simulink model "dual_single_phase_parallel_inverter_r2024a"  (R2024a)
settings: Solver=ode23t  StartTime=0.0  StopTime=0.25  MaxStep=5e-6  RelTol=1e-4
model workspace (MAT data in the model file):
  Paux1_W = 1
  Paux2_W = 1
libraries: nesl_utility x41, fl_lib x39, ee_lib x31, simulink x6
(part 4 of 4)

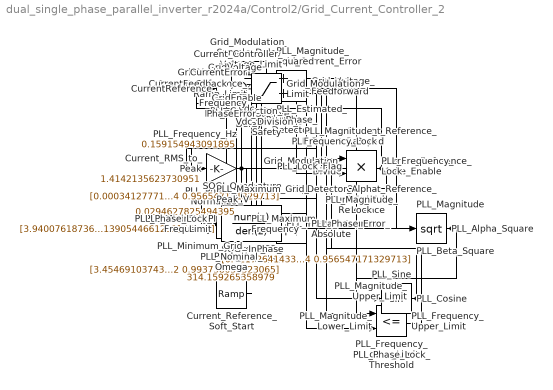
== system dual_single_phase_parallel_inverter_r2024a/Control2/Grid_Current_Controller_2 ==
  GridVoltage : Inport
  IrefRms : Inport  Port=2
  CurrentFeedback : Inport  Port=3
  Vdc : Inport  Port=4
  GridEnable : Inport  Port=5
  Current_Controller_Voltage_Limit : Saturate  UpperLimit=16  LowerLimit=-16
  Current_PR_Controller : DiscreteTransferFcn  Numerator=[3.45469103743655 -6.26042259834152 2.80882171809216]  Denominator=[1 -1.99275440474052 0.993738032323065]  SampleTime=1e-4
  Current_RMS_to_Peak : Gain  Gain=1.4142135623730951
  Current_Reference_Mode_Enable : Product
  Current_Reference_PLL_Lock : Product
  Current_Reference_Ramp_Limit : Saturate  UpperLimit=1  LowerLimit=0
  Current_Reference_Ramped : Product
  Current_Reference_Soft_Start : simulink/Sources/Ramp  slope=5  start=0  InitialOutput=0
  Current_Sine_Reference : Product
  Grid_Current_Error : Sum  Inputs=+-
  Grid_Modulation_Divide : Product  Inputs=*/
  Grid_Modulation_Limit : Saturate  UpperLimit=0.95  LowerLimit=-0.95
  Grid_Modulation_Sample_Delay : UnitDelay  SampleTime=1e-4  HasFrameUpgradeWarning=on
  Grid_Voltage_Feedforward : Sum
  PLL_Alpha_Square : Math  Operator=square
  PLL_Beta_Square : Math  Operator=square
  PLL_Correction_Limit : Saturate  UpperLimit=31.4159265359  LowerLimit=-31.4159265359
  PLL_Cosine : Trigonometry  Operator=cos
  PLL_Detector_Alpha : Product
  PLL_Detector_Beta : Product
  PLL_Estimated_Omega : Sum
  PLL_Frequency_Hz : Gain  Gain=0.159154943091895
  PLL_Frequency_Lock : Product
  PLL_Frequency_Lower_Limit : RelationalOperator  OutDataTypeStr=boolean  RndMeth=Simplest  InputSameDT=off
  PLL_Frequency_Upper_Limit : RelationalOperator  Operator=<=  OutDataTypeStr=boolean  RndMeth=Simplest  InputSameDT=off
  PLL_Lock_Flag : Product
  PLL_Magnitude : Math  Operator=sqrt
  PLL_Magnitude_Frequency_Lock : Product
  PLL_Magnitude_Lock : Product
  PLL_Magnitude_Lower_Limit : RelationalOperator  OutDataTypeStr=boolean  RndMeth=Simplest  InputSameDT=off
  PLL_Magnitude_Squared : Sum
  PLL_Magnitude_Upper_Limit : RelationalOperator  Operator=<=  OutDataTypeStr=boolean  RndMeth=Simplest  InputSameDT=off
  PLL_Maximum_Frequency : Constant  Value=50.5
  PLL_Maximum_Grid_Peak_V : Constant  Value=48
  PLL_Minimum_Frequency : Constant  Value=49.5
  PLL_Minimum_Grid_Peak_V : Constant  Value=20
  PLL_Nominal_Omega : Constant  Value=314.159265358979
  PLL_PI : DiscreteTransferFcn  Numerator=[3.94007618736156 -3.91390544661292]  Denominator=[1 -1]  SampleTime=1e-4
  PLL_Phase_Detector : Sum
  PLL_Phase_Error_Absolute : Abs  SaturateOnIntegerOverflow=off
  PLL_Phase_Lock_Limit : Constant  Value=0.05
  PLL_Phase_Lock_Threshold : RelationalOperator  Operator=<=  OutDataTypeStr=boolean  RndMeth=Simplest  InputSameDT=off
  PLL_Phase_Normalize : Gain  Gain=0.0294627825494395
  PLL_Sine : Trigonometry
  PLL_Theta_Integrator : DiscreteTransferFcn  Numerator=[1e-4 0]  Denominator=[1 -1]  SampleTime=1e-4
  PLL_Theta_Sample_Delay : UnitDelay  SampleTime=1e-4  HasFrameUpgradeWarning=on
  SOGI_InPhase : DiscreteTransferFcn  Numerator=[0.0217264143351434 0 -0.0217264143351434]  Denominator=[1 -1.95558189217414 0.956547171329713]  SampleTime=1e-4
  SOGI_Quadrature : DiscreteTransferFcn  Numerator=[0.000341277718320673 0.000682555436641346 0.000341277718320673]  Denominator=[1 -1.95558189217414 0.956547171329713]  SampleTime=1e-4
  Vdc_Division_Safety : Saturate  UpperLimit=100  LowerLimit=1
  GridModulation : Outport
  Theta : Outport  Port=2
  Frequency : Outport  Port=3
  Lock : Outport  Port=4
  CurrentReference : Outport  Port=5
  CurrentError : Outport  Port=6
  PhaseError : Outport  Port=7
  wires:
  GridVoltage/1 -> SOGI_InPhase/1, SOGI_Quadrature/1, Grid_Voltage_Feedforward/2
  SOGI_InPhase/1 -> PLL_Detector_Alpha/1, PLL_Alpha_Square/1
  PLL_Cosine/1 -> PLL_Detector_Alpha/2
  SOGI_Quadrature/1 -> PLL_Detector_Beta/1, PLL_Beta_Square/1
  PLL_Sine/1 -> PLL_Detector_Beta/2, Current_Sine_Reference/2
  PLL_Detector_Alpha/1 -> PLL_Phase_Detector/1
  PLL_Detector_Beta/1 -> PLL_Phase_Detector/2
  PLL_Phase_Detector/1 -> PLL_Phase_Normalize/1
  PLL_Phase_Normalize/1 -> PLL_PI/1, PhaseError/1, PLL_Phase_Error_Absolute/1
  PLL_PI/1 -> PLL_Correction_Limit/1
  PLL_Correction_Limit/1 -> PLL_Estimated_Omega/1
  PLL_Nominal_Omega/1 -> PLL_Estimated_Omega/2
  PLL_Estimated_Omega/1 -> PLL_Theta_Integrator/1, PLL_Frequency_Hz/1
  PLL_Frequency_Hz/1 -> Frequency/1, PLL_Frequency_Lower_Limit/1, PLL_Frequency_Upper_Limit/1
  PLL_Minimum_Frequency/1 -> PLL_Frequency_Lower_Limit/2
  PLL_Maximum_Frequency/1 -> PLL_Frequency_Upper_Limit/2
  PLL_Phase_Error_Absolute/1 -> PLL_Phase_Lock_Threshold/1
  PLL_Phase_Lock_Limit/1 -> PLL_Phase_Lock_Threshold/2
  PLL_Alpha_Square/1 -> PLL_Magnitude_Squared/1
  PLL_Beta_Square/1 -> PLL_Magnitude_Squared/2
  PLL_Magnitude_Squared/1 -> PLL_Magnitude/1
  PLL_Magnitude/1 -> PLL_Magnitude_Lower_Limit/1, PLL_Magnitude_Upper_Limit/1
  PLL_Minimum_Grid_Peak_V/1 -> PLL_Magnitude_Lower_Limit/2
  PLL_Maximum_Grid_Peak_V/1 -> PLL_Magnitude_Upper_Limit/2
  PLL_Magnitude_Lower_Limit/1 -> PLL_Magnitude_Lock/1
  PLL_Magnitude_Upper_Limit/1 -> PLL_Magnitude_Lock/2
  PLL_Frequency_Lower_Limit/1 -> PLL_Frequency_Lock/1
  PLL_Frequency_Upper_Limit/1 -> PLL_Frequency_Lock/2
  PLL_Magnitude_Lock/1 -> PLL_Magnitude_Frequency_Lock/1
  PLL_Frequency_Lock/1 -> PLL_Magnitude_Frequency_Lock/2
  PLL_Magnitude_Frequency_Lock/1 -> PLL_Lock_Flag/1
  PLL_Phase_Lock_Threshold/1 -> PLL_Lock_Flag/2
  PLL_Lock_Flag/1 -> Lock/1, Current_Reference_PLL_Lock/2
  IrefRms/1 -> Current_RMS_to_Peak/1
  Current_RMS_to_Peak/1 -> Current_Sine_Reference/1
  Current_Reference_Soft_Start/1 -> Current_Reference_Ramp_Limit/1
  Current_Sine_Reference/1 -> Current_Reference_Ramped/1
  Current_Reference_Ramp_Limit/1 -> Current_Reference_Ramped/2
  Current_Reference_Ramped/1 -> Current_Reference_Mode_Enable/1
  GridEnable/1 -> Current_Reference_Mode_Enable/2
  Current_Reference_Mode_Enable/1 -> Current_Reference_PLL_Lock/1
  Current_Reference_PLL_Lock/1 -> CurrentReference/1, Grid_Current_Error/1
  CurrentFeedback/1 -> Grid_Current_Error/2
  Grid_Current_Error/1 -> CurrentError/1, Current_PR_Controller/1
  Current_PR_Controller/1 -> Current_Controller_Voltage_Limit/1
  Current_Controller_Voltage_Limit/1 -> Grid_Voltage_Feedforward/1
  Grid_Voltage_Feedforward/1 -> Grid_Modulation_Divide/1
  Vdc/1 -> Vdc_Division_Safety/1
  Vdc_Division_Safety/1 -> Grid_Modulation_Divide/2
  Grid_Modulation_Divide/1 -> Grid_Modulation_Limit/1
  Grid_Modulation_Limit/1 -> Grid_Modulation_Sample_Delay/1
  Grid_Modulation_Sample_Delay/1 -> GridModulation/1
  PLL_Theta_Integrator/1 -> PLL_Theta_Sample_Delay/1
  PLL_Theta_Sample_Delay/1 -> PLL_Sine/1, PLL_Cosine/1, Theta/1
